simulink library "carnot"  (R2013b)
settings: Solver=ode45  StartTime=0.0  StopTime=10.0  RelTol=1e-3
undefined symbols (not defined in the file or in its folder): A, acol, Ahabit, Awin, Azimuth_Angle, AziWin, B, C, c1, c4, capc, caph, CarnotCallbacks_Density, CarnotCallbacks_Enthalpy, CarnotCallbacks_Enthalpy2Temperature, CarnotCallbacks_Entropy, CarnotCallbacks_Evaporation_Enthalpy, CarnotCallbacks_GlobalMessageLevel, CarnotCallbacks_Grashof, CarnotCallbacks_Heat_Capacity, CarnotCallbacks_Kinematic_Viscosity, CarnotCallbacks_Prandtl, CarnotCallbacks_Saturation_Property, CarnotCallbacks_Saturation_Temperature, CarnotCallbacks_Saturation_Value_Water, CarnotCallbacks_Specific_Volume, CarnotCallbacks_Thermal_Conductivity, CarnotCallbacks_Vapour_Content, CarnotCallbacks_Vapour_Pressure, con, cond, d, Dd, density, dfin, dia, DiameterLastPiece, DPConstant, dpipe, DPLinear, DPQuadratic, emission_out, fluid, FluidMix, FluidType, FPC, frame, g, GeodeticHeight, Gwin, heat_capacity, hgt, HP, Hroom, ID, inlet, K, l, lin, lpipe ... (+29)
undefined symbols (not defined in the file): c2, c3, c5, c6, cwall, dactive, height, mc, mID, rho, tau, UAneighbour, UAwall, uloss
libraries: carnot x333, simulink x25, simulink_extras x7
(part 15 of 16)

== system carnot/Source/Ventilation/Ventilation_AIV/Subsystem ==
  note: (kg/s)
  note: (kg/s)
  note: (kg/s)
  note: (kg/kg)
  note: (kg/kg)
  note: ASSUMPTION: mdot_air_out2in = mdot_air_in2out !
  mdot_air : Inport
  x_in : Inport  Port=2
  x_out : Inport  Port=3
  Demux2 : Demux  Outputs=2
  Demux3 : Demux  Outputs=2
  Fcn{,1..3} (4 alike) : Fcn  Expr=u / (1+u)
  Product5 : Product  SaturateOnIntegerOverflow=on  InputSameDT=on  OutDataTypeStr=Inherit: Same as first input
  Product6 : Product  SaturateOnIntegerOverflow=on  InputSameDT=on  OutDataTypeStr=Inherit: Same as first input
  Sum1 : Sum  Inputs=+-  SaturateOnIntegerOverflow=on  InputSameDT=on  OutDataTypeStr=Inherit: Same as first input
  Sum2 : Sum  Inputs=+-  SaturateOnIntegerOverflow=on  InputSameDT=on  OutDataTypeStr=Inherit: Same as first input
  mdot_H2O : Outport
  mdot_CO2 : Outport  Port=2
  wires:
  x_out/1 -> Demux2/1
  Demux2/1 -> Fcn/1  "x_H2O_out"
  Demux2/2 -> Fcn1/1  "x_CO2_out"
  Demux3/2 -> Fcn3/1  "x_CO2_in"
  Demux3/1 -> Fcn2/1  "x_H2O_in"
  x_in/1 -> Demux3/1
  Fcn/1 -> Sum1/1
  Fcn2/1 -> Sum1/2
  Fcn1/1 -> Sum2/1
  Fcn3/1 -> Sum2/2
  Sum2/1 -> Product6/2
  Sum1/1 -> Product5/2
  mdot_air/1 -> Product6/1, Product5/1  "mdot_air >=0"
  Product6/1 -> mdot_CO2/1
  Product5/1 -> mdot_H2O/1

== system carnot/Storage/Thermal/Storage_Ports/Electric_Heating ==
  electric power : Inport
  Gain : Gain  Gain=Q
  Mux3 : Mux  Inputs=8
  T_in : Constant  Value=ones(nodes,1)*20
  const2 : Constant  Value=1e5
  const3 : Constant
  const4 : Constant  Value=0
  mdot : Constant  Value=zeros(nodes,1)
  to_storeT : Outport
  wires:
  const3/1 -> Mux3/7
  const2/1 -> Mux3/6
  mdot/1 -> Mux3/2, Mux3/3, Mux3/4  "mdot_in"
  Mux3/1 -> to_storeT/1
  T_in/1 -> Mux3/1  "T_in"
  electric power/1 -> Gain/1
  const4/1 -> Mux3/8
  Gain/1 -> Mux3/5  "Qdot_in"

== system carnot/Storage/Thermal/Storage_Ports/HX_EN12977 ==
  from_storeT : Inport
  THBin : Inport  Port=2
  Bus Assignment1 : BusAssignment  AssignedSignals=Temperature
  Mux3 : Mux  Inputs=8
  Pressure_Drop_StorageHX : carnot/Basic/Pressure_Drop/Pressure_Drop_StorageHX  dia=dia  hgt=hgt
  T_in : Constant  Value=zeros(nodes,1)
  fluid : Constant  Value=-9999
  mdot_in : Constant  Value=zeros(nodes,1)
  mix : Constant  Value=-9999
  p : Constant  Value=-9999
  select_Tout : Selector  InputPortWidth=nodes  IndexOptions=Index vector (dialog)  Indices=[outlet]  OutputSizes=1
  sfun_storage_heatexchanger : carnot/Basic/Thermal_Models/sfun_storage_heatexchanger  idn=heat transfer data fit EN12977  nodes=nodes  inlet=inlet  outlet=outlet  pp=[ua0, uam, uat, 0,0,0,0]
  to_storeT : Outport  InitialOutput=0
  THBout : Outport  Port=2  InitialOutput=0
  wires:
  from_storeT/1 -> sfun_storage_heatexchanger/1
  THBin/1 -> Pressure_Drop_StorageHX/1, sfun_storage_heatexchanger/2
  mdot_in/1 -> Mux3/2, Mux3/3, Mux3/4  "mdot_in"
  Mux3/1 -> to_storeT/1
  select_Tout/1 -> Bus Assignment1/2
  T_in/1 -> Mux3/1  "T_in"
  sfun_storage_heatexchanger/1 -> Mux3/5  "Q_in"
  Bus Assignment1/1 -> THBout/1
  p/1 -> Mux3/6
  fluid/1 -> Mux3/7
  mix/1 -> Mux3/8
  sfun_storage_heatexchanger/2 -> select_Tout/1
  Pressure_Drop_StorageHX/1 -> Bus Assignment1/1

== system carnot/Storage/Thermal/Storage_Ports/HX_EN12977_stratified ==
  from_storeT : Inport
  THBin : Inport  Port=2
  Bus Assignment1 : BusAssignment  AssignedSignals=Temperature
  Mux3 : Mux  Inputs=8
  Pressure_Drop_StorageHX : carnot/Basic/Pressure_Drop/Pressure_Drop_StorageHX  dia=dia  hgt=hgt
  T_in : Constant  Value=zeros(nodes,1)
  fluid : Constant  Value=-9999
  mdot_in : Constant  Value=zeros(nodes,1)
  mix : Constant  Value=-9999
  p : Constant  Value=-9999
  select_Tout : Selector  InputPortWidth=nodes  IndexOptions=Index vector (dialog)  Indices=[outlet]  OutputSizes=1
  sfun_storage_heatexchanger : carnot/Basic/Thermal_Models/sfun_storage_heatexchanger  idn="heat transfer data fit EN12977  - stratified"  nodes=nodes  inlet=inlet  outlet=outlet  pp=[ua0, uam, uat, 0,0,0,0]
  to_storeT : Outport  InitialOutput=0
  THBout : Outport  Port=2  InitialOutput=0
  wires:
  from_storeT/1 -> sfun_storage_heatexchanger/1
  THBin/1 -> Pressure_Drop_StorageHX/1, sfun_storage_heatexchanger/2
  mdot_in/1 -> Mux3/2, Mux3/3, Mux3/4  "mdot_in"
  Mux3/1 -> to_storeT/1
  select_Tout/1 -> Bus Assignment1/2
  T_in/1 -> Mux3/1  "T_in"
  sfun_storage_heatexchanger/1 -> Mux3/5  "Q_in"
  Bus Assignment1/1 -> THBout/1
  p/1 -> Mux3/6
  fluid/1 -> Mux3/7
  mix/1 -> Mux3/8
  sfun_storage_heatexchanger/2 -> select_Tout/1
  Pressure_Drop_StorageHX/1 -> Bus Assignment1/1

== system carnot/Storage/Thermal/Storage_Ports/HX_data_fit ==
  note: UA = uac + mdot*uam + (Thx-Tstorage)*uat
      | Qdot = UA * (Tstore-Thx)
  from_storeT : Inport
  THBin : Inport  Port=2
  Bus Assignment1 : BusAssignment  AssignedSignals=Temperature
  Mux3 : Mux  Inputs=8
  Pressure_Drop_StorageHX : carnot/Basic/Pressure_Drop/Pressure_Drop_StorageHX  dia=dia  hgt=hgt
  T_in : Constant  Value=zeros(nodes,1)
  fluid : Constant  Value=-9999
  mdot_in : Constant  Value=zeros(nodes,1)
  mix : Constant  Value=-9999
  p : Constant  Value=-9999
  select_Tout : Selector  InputPortWidth=nodes  IndexOptions=Index vector (dialog)  Indices=[outlet]  OutputSizes=1
  sfun_storage_heatexchanger : carnot/Basic/Thermal_Models/sfun_storage_heatexchanger  idn=heat transfer from data fit  nodes=nodes  inlet=inlet  outlet=outlet  pp=[ua0, uam, uat, 0,0,0,0]
  to_storeT : Outport
  THBout : Outport  Port=2
  wires:
  sfun_storage_heatexchanger/2 -> select_Tout/1
  mix/1 -> Mux3/8
  fluid/1 -> Mux3/7
  p/1 -> Mux3/6
  Bus Assignment1/1 -> THBout/1
  sfun_storage_heatexchanger/1 -> Mux3/5  "Q_in"
  T_in/1 -> Mux3/1  "T_in"
  select_Tout/1 -> Bus Assignment1/2
  Mux3/1 -> to_storeT/1
  mdot_in/1 -> Mux3/4, Mux3/3, Mux3/2  "mdot_in"
  THBin/1 -> Pressure_Drop_StorageHX/1, sfun_storage_heatexchanger/2
  from_storeT/1 -> sfun_storage_heatexchanger/1
  Pressure_Drop_StorageHX/1 -> Bus Assignment1/1

== system carnot/Storage/Thermal/Storage_Ports/HX_data_fit_stratified ==
  note: statified charging !
      | heat transfer:
      | UA = uac + mdot*uam + (Thx-Tstorage)*uat
      | Qdot = UA * (Tstore-Thx)
  from_storeT : Inport
  THBin : Inport  Port=2
  Bus Assignment1 : BusAssignment  AssignedSignals=Temperature
  Mux3 : Mux  Inputs=8
  Pressure_Drop_StorageHX : carnot/Basic/Pressure_Drop/Pressure_Drop_StorageHX  dia=dia  hgt=hgt
  T_in : Constant  Value=zeros(nodes,1)
  fluid : Constant  Value=-9999
  mdot_in : Constant  Value=zeros(nodes,1)
  mix : Constant  Value=-9999
  p : Constant  Value=-9999
  select_Tout : Selector  InputPortWidth=nodes  IndexOptions=Index vector (dialog)  Indices=[outlet]  OutputSizes=1
  sfun_storage_heatexchanger : carnot/Basic/Thermal_Models/sfun_storage_heatexchanger  idn="heat transfer from data fit  - stratified"  nodes=nodes  inlet=inlet  outlet=outlet  pp=[ua0, uam, uat, 0,0,0,0]
  to_storeT : Outport  InitialOutput=0
  THBout : Outport  Port=2  InitialOutput=0
  wires:
  from_storeT/1 -> sfun_storage_heatexchanger/1
  THBin/1 -> Pressure_Drop_StorageHX/1, sfun_storage_heatexchanger/2
  mdot_in/1 -> Mux3/2, Mux3/3, Mux3/4  "mdot_in"
  Mux3/1 -> to_storeT/1
  select_Tout/1 -> Bus Assignment1/2
  T_in/1 -> Mux3/1  "T_in"
  sfun_storage_heatexchanger/1 -> Mux3/5  "Q_in"
  p/1 -> Mux3/6
  fluid/1 -> Mux3/7
  mix/1 -> Mux3/8
  sfun_storage_heatexchanger/2 -> select_Tout/1
  Pressure_Drop_StorageHX/1 -> Bus Assignment1/1
  Bus Assignment1/1 -> THBout/1

== system carnot/Storage/Thermal/Storage_Ports/HX_finned_tube ==
  from_storeT : Inport
  THBin : Inport  Port=2
  Bus Assignment1 : BusAssignment  AssignedSignals=Temperature
  Mux3 : Mux  Inputs=8
  Pressure_Drop_StorageHX : carnot/Basic/Pressure_Drop/Pressure_Drop_StorageHX  dia=dia  hgt=hgt
  T_in : Constant  Value=zeros(nodes,1)
  fluid : Constant  Value=-9999
  mdot_in : Constant  Value=zeros(nodes,1)
  mix : Constant  Value=-9999
  p : Constant  Value=-9999
  select_Tout : Selector  InputPortWidth=nodes  IndexOptions=Index vector (dialog)  Indices=[outlet]  OutputSizes=1
  sfun_storage_heatexchanger : carnot/Basic/Thermal_Models/sfun_storage_heatexchanger  idn=finned tube theoretical  nodes=nodes  inlet=inlet  outlet=outlet  pp=[dpipe, swall, lpipe, cond, dfin, sfin, nfin]
  to_storeT : Outport  InitialOutput=0
  THBout : Outport  Port=2  InitialOutput=0
  wires:
  from_storeT/1 -> sfun_storage_heatexchanger/1
  THBin/1 -> Pressure_Drop_StorageHX/1, sfun_storage_heatexchanger/2
  mdot_in/1 -> Mux3/2, Mux3/3, Mux3/4  "mdot_in"
  Mux3/1 -> to_storeT/1
  select_Tout/1 -> Bus Assignment1/2
  T_in/1 -> Mux3/1  "T_in"
  sfun_storage_heatexchanger/1 -> Mux3/5  "Q_in"
  Bus Assignment1/1 -> THBout/1
  p/1 -> Mux3/6
  fluid/1 -> Mux3/7
  mix/1 -> Mux3/8
  sfun_storage_heatexchanger/2 -> select_Tout/1
  Pressure_Drop_StorageHX/1 -> Bus Assignment1/1

== system carnot/Storage/Thermal/Storage_Ports/HX_finned_tube_stratified ==
  from_storeT : Inport
  THBin : Inport  Port=2
  Bus Assignment1 : BusAssignment  AssignedSignals=Temperature
  Mux3 : Mux  Inputs=8
  Pressure_Drop_StorageHX : carnot/Basic/Pressure_Drop/Pressure_Drop_StorageHX  dia=dia  hgt=hgt
  T_in : Constant  Value=zeros(nodes,1)
  fluid : Constant  Value=-9999
  mdot_in : Constant  Value=zeros(nodes,1)
  mix : Constant  Value=-9999
  p : Constant  Value=-9999
  select_Tout : Selector  InputPortWidth=nodes  IndexOptions=Index vector (dialog)  Indices=[outlet]  OutputSizes=1
  sfun_storage_heatexchanger : carnot/Basic/Thermal_Models/sfun_storage_heatexchanger  idn="finned tube theoretical  - stratified"  nodes=nodes  inlet=inlet  outlet=outlet  pp=[dpipe, swall, lpipe, cond, dfin, sfin, nfin]
  to_storeT : Outport  InitialOutput=0
  THBout : Outport  Port=2  InitialOutput=0
  wires:
  Pressure_Drop_StorageHX/1 -> Bus Assignment1/1
  sfun_storage_heatexchanger/2 -> select_Tout/1
  mix/1 -> Mux3/8
  fluid/1 -> Mux3/7
  p/1 -> Mux3/6
  Bus Assignment1/1 -> THBout/1
  sfun_storage_heatexchanger/1 -> Mux3/5  "Q_in"
  T_in/1 -> Mux3/1  "T_in"
  select_Tout/1 -> Bus Assignment1/2
  Mux3/1 -> to_storeT/1
  mdot_in/1 -> Mux3/4, Mux3/3, Mux3/2  "mdot_in"
  THBin/1 -> sfun_storage_heatexchanger/2, Pressure_Drop_StorageHX/1
  from_storeT/1 -> sfun_storage_heatexchanger/1

== system carnot/Storage/Thermal/Storage_Ports/HX_tube ==
  from_storeT : Inport
  THBin : Inport  Port=2
  Bus Assignment1 : BusAssignment  AssignedSignals=Temperature
  Mux3 : Mux  Inputs=8
  Pressure_Drop_StorageHX : carnot/Basic/Pressure_Drop/Pressure_Drop_StorageHX  dia=dia  hgt=hgt
  T_in : Constant  Value=zeros(nodes,1)
  fluid : Constant  Value=-9999
  mdot_in : Constant  Value=zeros(nodes,1)
  mix : Constant  Value=-9999
  p : Constant  Value=-9999
  select_Tout : Selector  InputPortWidth=nodes  IndexOptions=Index vector (dialog)  Indices=[outlet]  OutputSizes=1
  sfun_storage_heatexchanger : carnot/Basic/Thermal_Models/sfun_storage_heatexchanger  idn=smooth tube theoretical  nodes=nodes  inlet=inlet  outlet=outlet  pp=[dpipe, swall, lpipe, cond, 0,0,0]
  to_storeT : Outport  InitialOutput=0
  THBout : Outport  Port=2  InitialOutput=0
  wires:
  Pressure_Drop_StorageHX/1 -> Bus Assignment1/1
  sfun_storage_heatexchanger/2 -> select_Tout/1
  mix/1 -> Mux3/8
  fluid/1 -> Mux3/7
  p/1 -> Mux3/6
  Bus Assignment1/1 -> THBout/1
  sfun_storage_heatexchanger/1 -> Mux3/5  "Q_in"
  T_in/1 -> Mux3/1  "T_in"
  select_Tout/1 -> Bus Assignment1/2
  Mux3/1 -> to_storeT/1
  mdot_in/1 -> Mux3/4, Mux3/3, Mux3/2  "mdot_in"
  THBin/1 -> Pressure_Drop_StorageHX/1, sfun_storage_heatexchanger/2
  from_storeT/1 -> sfun_storage_heatexchanger/1

== system carnot/Storage/Thermal/Storage_Ports/HX_tube_stratified ==
  from_storeT : Inport
  THBin : Inport  Port=2
  Bus Assignment1 : BusAssignment  AssignedSignals=Temperature
  Mux3 : Mux  Inputs=8
  Pressure_Drop_StorageHX : carnot/Basic/Pressure_Drop/Pressure_Drop_StorageHX  dia=dia  hgt=hgt
  T_in : Constant  Value=zeros(nodes,1)
  fluid : Constant  Value=-9999
  mdot_in : Constant  Value=zeros(nodes,1)
  mix : Constant  Value=-9999
  p : Constant  Value=-9999
  select_Tout : Selector  InputPortWidth=nodes  IndexOptions=Index vector (dialog)  Indices=[outlet]  OutputSizes=1
  sfun_storage_heatexchanger : carnot/Basic/Thermal_Models/sfun_storage_heatexchanger  idn=smooth tube theoretical - stratified  nodes=nodes  inlet=inlet  outlet=outlet  pp=[dpipe, swall, lpipe, cond, 0,0,0]
  to_storeT : Outport  InitialOutput=0
  THBout : Outport  Port=2  InitialOutput=0
  wires:
  Pressure_Drop_StorageHX/1 -> Bus Assignment1/1
  sfun_storage_heatexchanger/2 -> select_Tout/1
  mix/1 -> Mux3/8
  fluid/1 -> Mux3/7
  p/1 -> Mux3/6
  Bus Assignment1/1 -> THBout/1
  sfun_storage_heatexchanger/1 -> Mux3/5  "Q_in"
  T_in/1 -> Mux3/1  "T_in"
  select_Tout/1 -> Bus Assignment1/2
  Mux3/1 -> to_storeT/1
  mdot_in/1 -> Mux3/4, Mux3/3, Mux3/2  "mdot_in"
  THBin/1 -> Pressure_Drop_StorageHX/1, sfun_storage_heatexchanger/2
  from_storeT/1 -> sfun_storage_heatexchanger/1

== system carnot/Storage/Thermal/Storage_Ports/Pipe ==
  from_storeT : Inport
  THBin : Inport  Port=2
  Bus Assignment : BusAssignment  AssignedSignals=Temperature
  Bus Selector : BusSelector  OutputSignals=Temperature,MassFlow,Pressure,FluidType,FluidMix
  Gain : Gain  Gain=in
  Gain1 : Gain  Gain=up
  Gain2 : Gain  Gain=down
  Gain3 : Gain  Gain=in
  Mux3 : Mux  Inputs=8
  Pressure_Drop_StoragePipe : carnot/Basic/Pressure_Drop/Pressure_Drop_StoragePipe  dia=dia  hgt=hgt
  Q_in : Constant  Value=zeros(nodes,1)
  select_Tin_2_Tout : Selector  InputPortWidth=nodes  IndexOptions=Index vector (dialog)  Indices=[idx_in_out]  OutputSizes=1
  select_Tout : Selector  InputPortWidth=nodes  IndexOptions=Index vector (dialog)  Indices=[outlet]  OutputSizes=1
  to_storeT : Outport
  THBout : Outport  Port=2
  wires:
  select_Tin_2_Tout/1 -> Pressure_Drop_StoragePipe/1
  Bus Selector/5 -> Mux3/8  "<FluidMix>"
  Bus Assignment/1 -> THBout/1
  Q_in/1 -> Mux3/5
  Gain3/1 -> Mux3/1  "T_in"
  select_Tout/1 -> Bus Assignment/2
  Mux3/1 -> to_storeT/1
  Gain2/1 -> Mux3/4  "mdot_down"
  Gain1/1 -> Mux3/3  "mdot_up"
  Gain/1 -> Mux3/2  "mdot_in"
  Bus Selector/1 -> Gain3/1  "<Temperature>"
  Bus Selector/2 -> Gain2/1, Gain1/1, Gain/1  "<MassFlow>"
  Bus Selector/3 -> Mux3/6  "<Pressure>"
  Bus Selector/4 -> Mux3/7  "<FluidType>"
  THBin/1 -> Bus Selector/1, Pressure_Drop_StoragePipe/2
  from_storeT/1 -> select_Tin_2_Tout/1, select_Tout/1
  Pressure_Drop_StoragePipe/1 -> Bus Assignment/1

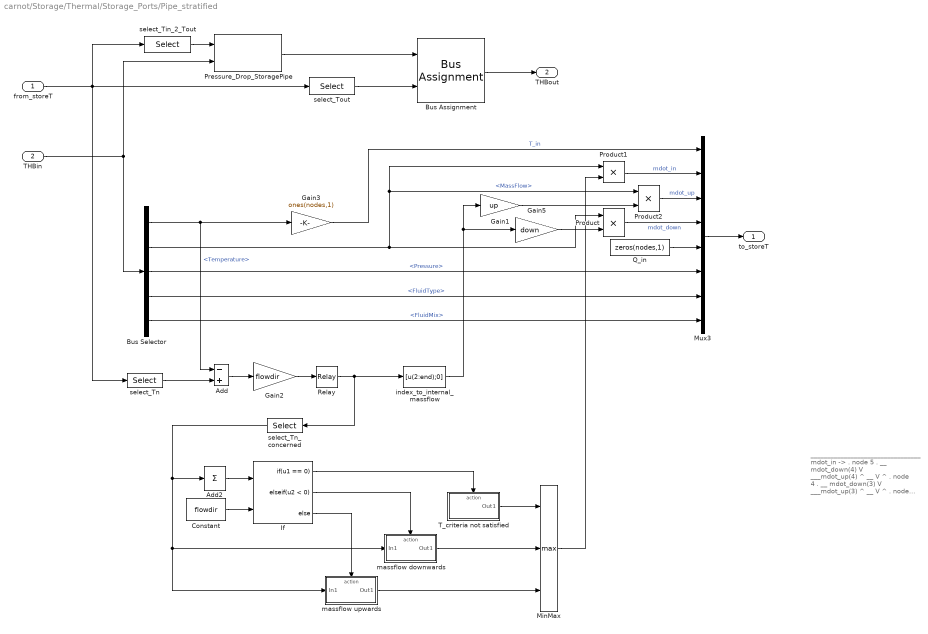
== system carnot/Storage/Thermal/Storage_Ports/Pipe_stratified ==
  note: _________________________________
      | mdot_in ->                                                .
      | node 5                     .
      | __ mdot_down(4) V  ___mdot_up(4) ^ __
      | V                           ^    .
      | node 4                    .
      | __ mdot_down(3) V  ___mdot_up(3) ^ __
      | V                           ^    .
      | node 3                    .
      | __ mdot_down(2) V  ___mdot_up(2) ^ __
      | V                           ^    .
      | node 2                    .
      | __ mdot_down(1) V  ___mdot_up(1) ^ __
      | V                           ^    .
      | node 1                    .
      | _________________________________
  from_storeT : Inport
  THBin : Inport  Port=2
  Add : Sum  Inputs=-+
  Add2 : Sum  Inputs=1
  Bus Assignment : BusAssignment  AssignedSignals=Temperature
  Bus Selector : BusSelector  OutputSignals=Temperature,MassFlow,Pressure,FluidType,FluidMix
  Constant : Constant  Value=flowdir
  Gain1 : Gain  Gain=up
  Gain2 : Gain  Gain=flowdir
  Gain3 : Gain  Gain=ones(nodes,1)
  Gain5 : Gain  Gain=down
  If : If  NumInputs=2  IfExpression=u1 == 0  ElseIfExpressions=u2 < 0
  MinMax : MinMax  Function=max  Inputs=3
  Mux3 : Mux  Inputs=8
  Pressure_Drop_StoragePipe : carnot/Basic/Pressure_Drop/Pressure_Drop_StoragePipe  dia=dia  hgt=hgt
  Product : Product  RndMeth=Zero
  Product1 : Product  RndMeth=Zero
  Product2 : Product  RndMeth=Zero
  Q_in : Constant  Value=zeros(nodes,1)
  Relay : Relay  OnSwitchValue=0.05  OffSwitchValue=-0.05
  T_criteria not satisfied : Subsystem  TreatAsAtomicUnit=on
  index_to_internal_massflow : MATLABFcn  MATLABFcn=[u(2:end);0]  OutputDimensions=nodes
  massflow downwards : Subsystem  TreatAsAtomicUnit=on
  massflow upwards : Subsystem  TreatAsAtomicUnit=on
  select_Tin_2_Tout : Selector  InputPortWidth=nodes  IndexOptions=Index vector (dialog)  Indices=[idx_in_out]  OutputSizes=1
  select_Tn : Selector  InputPortWidth=nodes  IndexOptions=Index vector (dialog)  Indices=[1:nodes]  OutputSizes=1
  select_Tn_concerned : Selector  InputPortWidth=nodes  IndexOptions=Index vector (dialog)  Indices=n_concerned  OutputSizes=1
  select_Tout : Selector  InputPortWidth=nodes  IndexOptions=Index vector (dialog)  Indices=[outlet]  OutputSizes=1
  to_storeT : Outport
  THBout : Outport  Port=2
  wires:
  select_Tin_2_Tout/1 -> Pressure_Drop_StoragePipe/1
  Pressure_Drop_StoragePipe/1 -> Bus Assignment/1
  select_Tn_concerned/1 -> Add2/1, massflow downwards/1(In1), massflow upwards/1(In1)
  MinMax/1 -> Product1/2
  Add2/1 -> If/1
  Product1/1 -> Mux3/2  "mdot_in"
  Gain5/1 -> Product/2
  Relay/1 -> select_Tn_concerned/1, index_to_internal_massflow/1
  Product/1 -> Mux3/4  "mdot_down"
  from_storeT/1 -> select_Tin_2_Tout/1, select_Tn/1, select_Tout/1
  THBin/1 -> Pressure_Drop_StoragePipe/2, Bus Selector/1
  Bus Selector/4 -> Mux3/7  "<FluidType>"
  Bus Selector/3 -> Mux3/6  "<Pressure>"
  Bus Selector/2 -> Product/1, Product2/1, Product1/1  "<MassFlow>"
  Bus Selector/1 -> Gain3/1, Add/1  "<Temperature>"
  Mux3/1 -> to_storeT/1
  select_Tout/1 -> Bus Assignment/2
  Gain3/1 -> Mux3/1  "T_in"
  Q_in/1 -> Mux3/5
  Bus Assignment/1 -> THBout/1
  Bus Selector/5 -> Mux3/8  "<FluidMix>"
  select_Tn/1 -> Add/2
  Add/1 -> Gain2/1
  If/1 -> T_criteria not satisfied/Action
  Constant/1 -> If/2
  T_criteria not satisfied/1(Out1) -> MinMax/1
  If/2 -> massflow downwards/Action
  If/3 -> massflow upwards/Action
  massflow downwards/1(Out1) -> MinMax/2
  Gain1/1 -> Product2/2
  Product2/1 -> Mux3/3  "mdot_up"
  massflow upwards/1(Out1) -> MinMax/3
  Gain2/1 -> Relay/1
  index_to_internal_massflow/1 -> Gain5/1, Gain1/1

== system carnot/Storage/Thermal/detailed_storage_models/heat_exchanger_storage ==
  Tamb : Inport
  THVex_in : Inport  Port=2
  THVstg_in : Inport  Port=3
  Demux : Demux
  Demux1 : Demux  Outputs=[1 1 1 1 2]
  Demux2 : Demux  Outputs=[1 1 1 1 2]
  Demux3 : Demux  Outputs=[6 14]
  Demux4 : Demux  Outputs=[6 14]
  Mux : Mux  Inputs=11
  Mux1 : Mux  Inputs=6
  Mux2 : Mux  Inputs=6
  S-Function : S-Function  FunctionName=ministg  Parameters=v(1), v(2), loss, uh(1), uh(2), uc(1), uc(2), uw(1), uw(2), mat, m(1), m(2), t0, dph(1), dph(2), dph(3), dpc(1), dpc(2), dpc(3), n  EnableBusSupport=off
  THVex : Outport
  THVstg : Outport  Port=2
  wires:
  Demux2/5 -> Mux2/5, Mux/11  "fluid, mix"
  Demux2/3 -> Mux2/3, Mux/9  "mdot"
  Demux1/5 -> Mux1/5, Mux/6  "fluid, mix"
  Demux1/3 -> Mux1/3, Mux/4  "mdot"
  Demux1/4 -> Mux/5
  Demux1/2 -> Mux/3
  Mux/1 -> S-Function/1
  Tamb/1 -> Mux/1
  Demux1/1 -> Mux1/1, Mux/2  "ID"
  Demux2/4 -> Mux/10
  Demux2/2 -> Mux/8
  Demux2/1 -> Mux2/1, Mux/7  "ID"
  S-Function/1 -> Demux/1
  Demux3/1 -> Demux1/1
  THVex_in/1 -> Demux3/1
  THVstg_in/1 -> Demux4/1
  Demux4/1 -> Demux2/1
  Demux/4 -> Mux2/4
  Demux/3 -> Mux2/2
  Mux2/1 -> THVstg/1
  Mux1/1 -> THVex/1
  Demux/2 -> Mux1/4
  Demux/1 -> Mux1/2
  Demux3/2 -> Mux1/6
  Demux4/2 -> Mux2/6

== system carnot/Storage/Thermal/surface_models/Isolated_Cover ==
  Tamb : Inport
  Mux2 : Mux  Inputs=2
  const1 : Constant  Value=[u 0]
  Tamb_utop_Iabs : Outport
  wires:
  Mux2/1 -> Tamb_utop_Iabs/1
  const1/1 -> Mux2/2
  Tamb/1 -> Mux2/1

== system carnot/Storage/Thermal/surface_models/Open_Surface ==
  WDB : Inport
  3*vwind : Gain  Gain=3  SaturateOnIntegerOverflow=on  OutDataTypeStr=Inherit: Same as input  ParamDataTypeStr=Inherit: Same as input
  Bus Selector : BusSelector  OutputSignals=Solar_Radiation_direct_surface,Solar_Radiation_diffuse_surface,Temperature_Ambient,Wind_Speed
  Fixed_Surface : carnot/Weather/Fixed_Surface  colangle=0  colazi=0  colrot=0
  Mux2 : Mux  Inputs=3
  Radiation_on_Inclined_Surface : carnot/Weather/Radiation_on_Inclined_Surface  sky=Perez 1990  reflect=0.2
  Sum : Sum  Inputs=2  SaturateOnIntegerOverflow=on  InputSameDT=on  OutDataTypeStr=Inherit: Same as first input
  add 5.6 : Subsystem  mask(add constant){c=5.6}
      mask prompts: c "constant c"
      mask help: This block adds a constant c to each element of the input vector.
      mask Help: file:///constant.htm
      mask Display: disp('+c');
  ground absorbtion : Gain  Gain=albedo  SaturateOnIntegerOverflow=on  OutDataTypeStr=Inherit: Same as input  ParamDataTypeStr=Inherit: Same as input
  Tamb_utop_Iabs : Outport
  wires:
  Bus Selector/2 -> Sum/2  "<Solar_Radiation_diffuse_surface>"
  WDB/1 -> Radiation_on_Inclined_Surface/1
  Fixed_Surface/1 -> Radiation_on_Inclined_Surface/2
  Radiation_on_Inclined_Surface/1 -> Bus Selector/1
  Bus Selector/3 -> Mux2/1  "<Temperature_Ambient>"
  ground absorbtion/1 -> Mux2/3
  Bus Selector/1 -> Sum/1  "<Solar_Radiation_direct_surface>"
  Sum/1 -> ground absorbtion/1
  3*vwind/1 -> add 5.6/1(In1)
  add 5.6/1(Out1) -> Mux2/2
  Mux2/1 -> Tamb_utop_Iabs/1
  Bus Selector/4 -> 3*vwind/1  "<Wind_Speed>"

== system carnot/Basic/Thermal_Models/Combustion_Calculation/exhaust gas/fluid//solid ==
  c : Inport
  h : Inport  Port=2
  s : Inport  Port=3
  n : Inport  Port=4
  w : Inport  Port=5
  Mux : Mux  Inputs=2
  Mux1 : Mux
  kgCO2 : Gain  Gain=3.67  SaturateOnIntegerOverflow=on  OutDataTypeStr=Inherit: Same as input  ParamDataTypeStr=Inherit: Same as input
  kgH2O : Fcn  Expr=9*u(1)+u(2)
  kgSO2 : Gain  Gain=2  SaturateOnIntegerOverflow=on  OutDataTypeStr=Inherit: Same as input  ParamDataTypeStr=Inherit: Same as input
  Out1 : Outport
  wires:
  n/1 -> Mux1/4
  s/1 -> kgSO2/1
  w/1 -> Mux/2
  Mux1/1 -> Out1/1
  h/1 -> Mux/1
  c/1 -> kgCO2/1
  kgSO2/1 -> Mux1/3
  kgH2O/1 -> Mux1/2
  kgCO2/1 -> Mux1/1
  Mux/1 -> kgH2O/1

== system carnot/Basic/Thermal_Models/Combustion_Calculation/exhaust gas/gas ==
  c : Inport
  h : Inport  Port=2
  s : Inport  Port=3
  n : Inport  Port=4
  Mux1 : Mux
  Terminator1 : Terminator
  kgCO2 : Gain  Gain=3.67  SaturateOnIntegerOverflow=on  OutDataTypeStr=Inherit: Same as input  ParamDataTypeStr=Inherit: Same as input
  kgH2O : Gain  Gain=9  SaturateOnIntegerOverflow=on  OutDataTypeStr=Inherit: Same as input  ParamDataTypeStr=Inherit: Same as input
  kgSO2 : Ground
  Out1 : Outport
  wires:
  n/1 -> Mux1/4
  kgSO2/1 -> Mux1/3
  kgH2O/1 -> Mux1/2
  kgCO2/1 -> Mux1/1
  Mux1/1 -> Out1/1
  s/1 -> Terminator1/1
  h/1 -> kgH2O/1
  c/1 -> kgCO2/1

== system carnot/Basic/Thermal_Models/HeatPump_basic/model cold side/add constant ==
  In1 : Inport
  Sum : Sum  SaturateOnIntegerOverflow=on  InputSameDT=on  OutDataTypeStr=Inherit: Same as first input
  const : Constant  Value=c
  Out1 : Outport
  wires:
  const/1 -> Sum/1
  In1/1 -> Sum/2
  Sum/1 -> Out1/1

== system carnot/Load/Houses/heat_transfer/alfa_wall_out/q rad ==
  note: Wall has a view on 50% ground and 50% sky (true for vertical walls).
      | Longwave radiation emissiviy of ground and sky assumed to be 1.
  Tamb : Inport
  Twall : Inport  Port=2
  Tsky : Inport  Port=3
  Bias : Bias  Bias=273.15
  Gain : Gain  Gain=[-1 0.5 0.5]*emission_out*5.67e-8
  Math Function : Math  Operator=square  SaturateOnIntegerOverflow=on
  Math Function1 : Math  Operator=square  SaturateOnIntegerOverflow=on
  Mux : Mux  Inputs=3
  Sum : Sum  Inputs=1  SaturateOnIntegerOverflow=on  InputSameDT=on  OutDataTypeStr=Inherit: Same as first input
  qrad : Outport
  wires:
  Math Function1/1 -> Gain/1
  Gain/1 -> Sum/1
  Math Function/1 -> Math Function1/1
  Mux/1 -> Bias/1
  Bias/1 -> Math Function/1
  Twall/1 -> Mux/1
  Sum/1 -> qrad/1
  Tamb/1 -> Mux/3
  Tsky/1 -> Mux/2

== system carnot/Load/Houses/heat_transfer/alfa_window_in/Irradiation into room ==
  note: Solar radiation into zone
  "[tau]" : Inport
  "[I_t]" : Inport  Port=2
  Dot Product : DotProduct  InputSameDT=on  OutDataTypeStr=Inherit: Inherit via internal rule
  Selector : Selector  InputPortWidth=3  IndexOptions=Index vector (dialog)  Indices=[1 3]  OutputSizes=1
  Sum2 : Sum  Inputs=1  SaturateOnIntegerOverflow=on  InputSameDT=on  OutDataTypeStr=Inherit: Same as first input
  const : Gain  Gain=gvalue  SaturateOnIntegerOverflow=on  OutDataTypeStr=Inherit: Same as input  ParamDataTypeStr=Inherit: Same as input
  qdot_sol : Outport
  wires:
  const/1 -> qdot_sol/1
  Sum2/1 -> const/1
  Dot Product/1 -> Sum2/1
  Selector/1 -> Dot Product/1
  "[tau]"/1 -> Selector/1  "tau_dir(teta), tau_dir(0), tau_dfu"
  "[I_t]"/1 -> Dot Product/2

== system carnot/Load/Houses/heat_transfer/alfa_window_in/transmission coefficient 1-2-3-4-layer(s) ==
  teta : Inport
  LUT_taualfa : Subsystem  mask(LOOK UP TABLE){}
      mask help:
      | This block delivers the standardized LIGHT TRANSMISSION COEFFICIENT of a window glass with 1, 2, 3 or 4 layers depending on the incidence angle. Each layer may be 3 to 8 mm thick.
      |
      | teta:    incidence angle = angle between surface normal and
      |                 incidence, degree
      | numlayer: number of layers within the window glass, [1,4].
      | tau:    transmission of glass layer stack, [0,1]
  Mux : Mux  Inputs=3
  numlayer : Constant  Value=numlayer
  perpendicular : Constant  Value=0
  tau,dfu - angle : Constant  Value=60
  "[tau]" : Outport
  wires:
  LUT_taualfa/1(tau) -> "[tau]"/1
  numlayer/1 -> LUT_taualfa/2(numlayer)
  Mux/1 -> LUT_taualfa/1(teta)
  perpendicular/1 -> Mux/2
  tau,dfu - angle/1 -> Mux/3
  teta/1 -> Mux/1

== system carnot/Load/Houses/room_nodes/Room_Node/Sensitive room temperature ==
  note: Sensitive temperature
  Tr : Inport
  Tc : Inport  Port=2
  1-share_c : Gain  Gain=1-share_c  SaturateOnIntegerOverflow=on  OutDataTypeStr=Inherit: Same as input  ParamDataTypeStr=Inherit: Same as input
  Sum : Sum  SaturateOnIntegerOverflow=on  InputSameDT=on  OutDataTypeStr=Inherit: Same as first input
  share_c : Gain  Gain=share_c  SaturateOnIntegerOverflow=on  OutDataTypeStr=Inherit: Same as input  ParamDataTypeStr=Inherit: Same as input
  Ts : Outport
  wires:
  Sum/1 -> Ts/1
  1-share_c/1 -> Sum/2  "Tr"
  share_c/1 -> Sum/1  "Tc"
  Tc/1 -> share_c/1
  Tr/1 -> 1-share_c/1

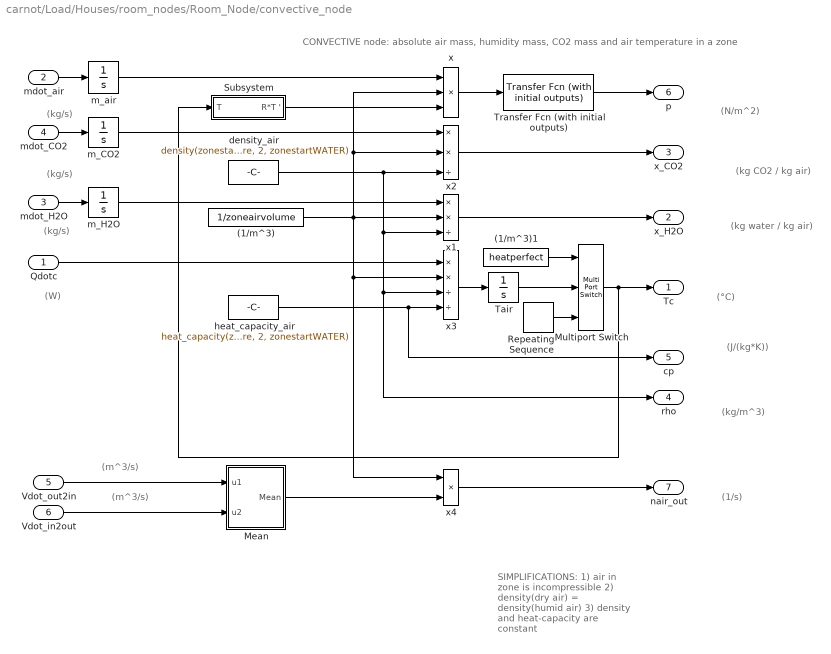
== system carnot/Load/Houses/room_nodes/Room_Node/convective_node ==
  note: (N/m^2)
  note: (kg CO2 / kg air)
  note: (J/(kg*K))
  note: SIMPLIFICATIONS:
      | 1) air in zone is incompressible
      | 2) density(dry air) = density(humid air)
      | 3) density and heat-capacity are constant
  note: (kg/m^3)
  note: CONVECTIVE node: absolute air mass, humidity mass, CO2 mass and air temperature in a zone
  note: (1/s)
  note: (m^3/s)
  note: (kg/s)
  note: (kg/s)
  note: (kg water / kg air)
  note: (°C)
  note: (W)
  note: (kg/s)
  note: (m^3/s)
  Qdotc : Inport
  mdot_air : Inport  Port=2
  mdot_H2O : Inport  Port=3
  mdot_CO2 : Inport  Port=4
  Vdot_out2in : Inport  Port=5
  Vdot_in2out : Inport  Port=6
  (1/m^3) : Constant  Value=1/zoneairvolume
  (1/m^3)1 : Constant  Value=heatperfect
  Mean : Subsystem
  Multiport Switch : MultiPortSwitch  Inputs=2  SaturateOnIntegerOverflow=on  InputSameDT=on
  Repeating Sequence : simulink/Sources/Repeating Sequence  rep_seq_t=lookuptime  rep_seq_y=lookupvalue
  Subsystem : Subsystem
  Tair : Integrator  InitialCondition=zonestartTEMP
  Transfer Fcn (with initial outputs) : simulink_extras/Additional Linear/Transfer Fcn (with initial outputs)  N=[1]  D=[timeconst 1]  Y0=1e5  U0=0
  density_air : Constant  Value=density(zonestartTEMP, AirPressure, 2, zonestartWATER)
  heat_capacity_air : Constant  Value=heat_capacity(zonestartTEMP, AirPressure, 2, zonestartWATER)
  m_CO2 : Integrator  InitialCondition=zonestartCO2  LimitOutput=on  LowerSaturationLimit=0
  m_H2O : Integrator  InitialCondition=zonestartWATER  LimitOutput=on  LowerSaturationLimit=0
  m_air : Integrator  InitialCondition=zonestartAIR  LimitOutput=on  LowerSaturationLimit=0
  x : Product  Inputs=***  SaturateOnIntegerOverflow=on  InputSameDT=on  OutDataTypeStr=Inherit: Same as first input
  x1 : Product  Inputs=**/  SaturateOnIntegerOverflow=on  InputSameDT=on  OutDataTypeStr=Inherit: Same as first input
  x2 : Product  Inputs=**/  SaturateOnIntegerOverflow=on  InputSameDT=on  OutDataTypeStr=Inherit: Same as first input
  x3 : Product  Inputs=**//  SaturateOnIntegerOverflow=on  InputSameDT=on  OutDataTypeStr=Inherit: Same as first input
  x4 : Product  Inputs=**  SaturateOnIntegerOverflow=on  InputSameDT=on  OutDataTypeStr=Inherit: Same as first input
  Tc : Outport
  x_H2O : Outport  Port=2
  x_CO2 : Outport  Port=3
  rho : Outport  Port=4
  cp : Outport  Port=5
  p : Outport  Port=6
  nair_out : Outport  Port=7
  wires:
  Repeating Sequence/1 -> Multiport Switch/3
  (1/m^3)1/1 -> Multiport Switch/1
  Multiport Switch/1 -> Tc/1, Subsystem/1(T)
  x2/1 -> x_CO2/1
  Tair/1 -> Multiport Switch/2
  x3/1 -> Tair/1
  (1/m^3)/1 -> x4/1, x3/2, x1/2, x/2, x2/2
  m_CO2/1 -> x2/1
  heat_capacity_air/1 -> cp/1, x3/4
  m_air/1 -> x/1
  mdot_air/1 -> m_air/1
  Subsystem/1(R*T ') -> x/3
  x1/1 -> x_H2O/1
  mdot_H2O/1 -> m_H2O/1
  mdot_CO2/1 -> m_CO2/1
  m_H2O/1 -> x1/1
  x/1 -> Transfer Fcn (with initial outputs)/1
  x4/1 -> nair_out/1
  Vdot_in2out/1 -> Mean/2(u2)
  Vdot_out2in/1 -> Mean/1(u1)
  Mean/1(Mean) -> x4/2
  Qdotc/1 -> x3/1
  density_air/1 -> x2/3, x1/3, x3/3, rho/1
  Transfer Fcn (with initial outputs)/1 -> p/1

== system carnot/Load/Houses/room_nodes/Room_Node/radiative_node ==
  note: RADIATIVE node
  Qdotr : Inport
  (1/m^3)1 : Constant  Value=heatperfect
  Gain : Gain  Gain=1/timeconst
  Integrator : Integrator  InitialCondition=zonestartTEMP
  Multiport Switch : MultiPortSwitch  Inputs=2  SaturateOnIntegerOverflow=on  InputSameDT=on
  Repeating Sequence : simulink/Sources/Repeating Sequence  rep_seq_t=lookuptime  rep_seq_y=lookupvalue
  Tr : Outport
  wires:
  Repeating Sequence/1 -> Multiport Switch/3
  Gain/1 -> Integrator/1
  Qdotr/1 -> Gain/1
  (1/m^3)1/1 -> Multiport Switch/1
  Integrator/1 -> Multiport Switch/2
  Multiport Switch/1 -> Tr/1

== system carnot/Load/Houses/wall_floor/Window_with_Shading/alfa_window_in ==
  note: (W/m^2)
  note: CONVENTION:
      | Qdot > 0 and qdots < 0, if Ts > T (heat flows from wall surface to room node),
      | Qdot < 0 and qdots > 0, if Ts < T (heat flows from room node to wall surface).
  note: s: surface
      | c: convective
      | r: radiative
  note: WINDOW = FRAME + GLASS
  note: Convective and radiative heat transfer at the INDOOR SURFACE OF A VERTICAL WINDOW
      | with 1-4 layers (each 3 ... 8 mm thick)
  note: (°C)
  Ts2 : Inport
  "[sun_t]" : Inport  Port=2
  "[AIV]" : Inport  Port=3
  WDB : Inport  Port=4
  control : Inport  Port=5
  Demux : Demux  Outputs=[1 1 1 6]
  Ground : Ground
  Ground1 : Ground
  Mux : Mux  Inputs=2
  Mux1 : Mux  Inputs=[1 5 2 5]
  Product5 : Product  SaturateOnIntegerOverflow=on  RndMeth=Zero  InputSameDT=on  OutDataTypeStr=Inherit: Same as first input
  Sum : Sum  Inputs=-+  SaturateOnIntegerOverflow=on  InputSameDT=on  OutDataTypeStr=Inherit: Same as first input
  Sum1 : Sum  Inputs=+-  SaturateOnIntegerOverflow=on  InputSameDT=on  OutDataTypeStr=Inherit: Same as first input
  Sum2 : Sum  Inputs=--+  SaturateOnIntegerOverflow=on  InputSameDT=on  OutDataTypeStr=Inherit: Same as first input
  Terminator : Terminator
  Terminator1 : Terminator
  emission_in : Gain  Gain=emission_in  SaturateOnIntegerOverflow=on  OutDataTypeStr=Inherit: Same as input  ParamDataTypeStr=Inherit: Same as input
  surface of window : Gain  Gain=windowsurface  SaturateOnIntegerOverflow=on  OutDataTypeStr=Inherit: Same as input  ParamDataTypeStr=Inherit: Same as input
  surface of window glass : Gain  Gain=(1-frame)*windowsurface  SaturateOnIntegerOverflow=on  OutDataTypeStr=Inherit: Same as input  ParamDataTypeStr=Inherit: Same as input
  transmission_absorption : Subsystem
  u_convection : Gain  Gain=2.5  SaturateOnIntegerOverflow=on  OutDataTypeStr=Inherit: Same as input  ParamDataTypeStr=Inherit: Same as input
  u_rad : Constant  Value=5.6
  qdots2 : Outport
  "[S]" : Outport  Port=2
  wires:
  Ground1/1 -> Mux1/4
  Ground/1 -> Mux1/2
  Mux1/1 -> "[S]"/1
  Sum2/1 -> qdots2/1
  Demux/4 -> Terminator1/1
  "[AIV]"/1 -> Demux/1
  Demux/1 -> Terminator/1
  Mux/1 -> surface of window/1
  emission_in/1 -> Product5/1
  Sum1/1 -> Product5/2  "dTr"
  u_rad/1 -> emission_in/1
  Ts2/1 -> Sum/2, Sum1/1  "Ts"
  Product5/1 -> Mux/2, Sum2/2  "qdotr"
  u_convection/1 -> Sum2/1, Mux/1  "qdotc"
  "[sun_t]"/1 -> transmission_absorption/1(sun_t)
  surface of window glass/1 -> Mux1/1  "Qdot_sol"
  surface of window/1 -> Mux1/3  "[Qdotc, Qdotr]"
  Demux/2 -> Sum/1  "Tc"
  Sum/1 -> u_convection/1  "dTc"
  Demux/3 -> Sum1/2  "Tr"
  transmission_absorption/2(qdot_sol) -> surface of window glass/1  "qdot_sol (> =0)"
  transmission_absorption/1(qdot_abs) -> Sum2/3  "qabs"
  WDB/1 -> transmission_absorption/2(WDB)
  control/1 -> transmission_absorption/3(control)

== system carnot/Load/Houses/wall_floor/Window_with_Shading/lambda_window ==
  note: Timeconstant of window is calculated
      | in the mask initialization
  note: Heat conduction in a window (ONLY SURFACE LAYER CONNECTABLE)
  qdots1 : Inport
  qdots2 : Inport  Port=2
  Product1 : Product  SaturateOnIntegerOverflow=on  RndMeth=Zero  InputSameDT=on  OutDataTypeStr=Inherit: Same as first input
  Product6 : Product  SaturateOnIntegerOverflow=on  RndMeth=Zero  InputSameDT=on  OutDataTypeStr=Inherit: Same as first input
  R_win : Constant  Value=Rwin
  Sum1 : Sum  SaturateOnIntegerOverflow=on  InputSameDT=on  OutDataTypeStr=Inherit: Same as first input
  Sum3 : Sum  SaturateOnIntegerOverflow=on  InputSameDT=on  OutDataTypeStr=Inherit: Same as first input
  Transfer Fcn : TransferFcn  Denominator=[timeconst 1]
  Transfer Fcn1 : TransferFcn  Denominator=[timeconst 1]
  Ts1 : Outport
  Ts2 : Outport  Port=2
  wires:
  R_win/1 -> Product1/1, Product6/1  "R_win"
  Sum1/1 -> Transfer Fcn1/1
  Product1/1 -> Sum1/1
  Sum3/1 -> Transfer Fcn/1
  Product6/1 -> Sum3/1
  qdots2/1 -> Product1/2
  qdots1/1 -> Product6/2
  Transfer Fcn/1 -> Sum1/2, Ts1/1
  Transfer Fcn1/1 -> Sum3/2, Ts2/1

== system carnot/Source/Chiller/Absorption_Chiller_ddT/absorber // condenser/Tcooler_out ==
  T : Inport
  mdot : Inport  Port=2
  Qdot_E + Qdot_G : Inport  Port=3
  p : Inport  Port=4
  fluid : Inport  Port=5
  mix : Inport  Port=6
  Heat_Capacity : carnot/Basic/Material_Properties/Heat_Capacity  VariantControl=CarlibClassic  INPUTARGUMENTS=state variables (classic)  DEBUGLEVEL=DEBUGLEVEL  MAXTOTALWARNINGS=inf  MAXCONSECUTIVEWARNINGS=inf  WRITETOFILE=0  FILENAME='errors.txt'
  Product1 : Product  Inputs=//*  SaturateOnIntegerOverflow=on  InputSameDT=on  OutDataTypeStr=Inherit: Same as first input
  Saturation : Saturate  UpperLimit=inf  LowerLimit=1e-5
  Sum3 : Sum  SaturateOnIntegerOverflow=on  InputSameDT=on  OutDataTypeStr=Inherit: Same as first input
  Tcooler_out : Outport  InitialOutput=0
  wires:
  Qdot_E + Qdot_G/1 -> Product1/3
  Saturation/1 -> Product1/1
  Sum3/1 -> Tcooler_out/1
  mdot/1 -> Saturation/1
  Product1/1 -> Sum3/2
  Heat_Capacity/1 -> Product1/2
  T/1 -> Heat_Capacity/1, Sum3/1
  p/1 -> Heat_Capacity/2
  fluid/1 -> Heat_Capacity/3
  mix/1 -> Heat_Capacity/4

== system carnot/Source/Chiller/Absorption_Chiller_ddT/boiler/Qdot_G with deltadelta_t ==
  deltadelta_t : Inport
  Add1 : Sum
  Constant : Constant  Value=rG
  Gain1 : Gain  Gain=sG
  Transfer Fcn : TransferFcn  Denominator=[600 1]
  kW_2_W : Gain  Gain=1000
  Qdot_G [W] : Outport
  wires:
  Transfer Fcn/1 -> Qdot_G [W]/1
  kW_2_W/1 -> Transfer Fcn/1
  Add1/1 -> kW_2_W/1
  deltadelta_t/1 -> Gain1/1
  Gain1/1 -> Add1/2
  Constant/1 -> Add1/1

== system carnot/Source/Chiller/Absorption_Chiller_ddT/boiler/Thot_out ==
  Thot_in : Inport
  mdot : Inport  Port=2
  Qdot_G : Inport  Port=3
  p : Inport  Port=4
  fluid : Inport  Port=5
  mix : Inport  Port=6
  Heat_Capacity : carnot/Basic/Material_Properties/Heat_Capacity  VariantControl=CarlibClassic  INPUTARGUMENTS=state variables (classic)  DEBUGLEVEL=DEBUGLEVEL  MAXTOTALWARNINGS=inf  MAXCONSECUTIVEWARNINGS=inf  WRITETOFILE=0  FILENAME='errors.txt'
  Product1 : Product  Inputs=//*  SaturateOnIntegerOverflow=on  InputSameDT=on  OutDataTypeStr=Inherit: Same as first input
  Saturation : Saturate  UpperLimit=inf  LowerLimit=1e-5
  Sum3 : Sum  Inputs=+-  SaturateOnIntegerOverflow=on  InputSameDT=on  OutDataTypeStr=Inherit: Same as first input
  Thot_out : Outport  InitialOutput=0
  wires:
  Qdot_G/1 -> Product1/3
  Saturation/1 -> Product1/1
  Sum3/1 -> Thot_out/1
  mdot/1 -> Saturation/1
  Product1/1 -> Sum3/2
  Heat_Capacity/1 -> Product1/2
  Thot_in/1 -> Heat_Capacity/1, Sum3/1
  p/1 -> Heat_Capacity/2
  fluid/1 -> Heat_Capacity/3
  mix/1 -> Heat_Capacity/4

== system carnot/Source/Chiller/Absorption_Chiller_ddT/evaporator/Qdot_E with deltadelta_t ==
  deltadelta_t : Inport
  Add1 : Sum
  Constant : Constant  Value=rE
  Gain1 : Gain  Gain=sE
  Transfer Fcn : TransferFcn  Denominator=[600 1]
  kW_2_W : Gain  Gain=1000
  Qdot_E [W] : Outport
  wires:
  Transfer Fcn/1 -> Qdot_E [W]/1
  kW_2_W/1 -> Transfer Fcn/1
  Add1/1 -> kW_2_W/1
  deltadelta_t/1 -> Gain1/1
  Gain1/1 -> Add1/2
  Constant/1 -> Add1/1

== system carnot/Source/Chiller/Absorption_Chiller_ddT/evaporator/Tchilled_out ==
  note: Qdot_chilled_out = Qdot_chilled_in - Q_E
      | tchilled_out = Tchilled_in * mdot* cp - Qdot_E / (mdot * cp)
  T : Inport
  mdot : Inport  Port=2
  Qdot_E : Inport  Port=3
  p : Inport  Port=4
  fluid : Inport  Port=5
  mix : Inport  Port=6
  Heat_Capacity : carnot/Basic/Material_Properties/Heat_Capacity  VariantControl=CarlibClassic  INPUTARGUMENTS=state variables (classic)  DEBUGLEVEL=DEBUGLEVEL  MAXTOTALWARNINGS=inf  MAXCONSECUTIVEWARNINGS=inf  WRITETOFILE=0  FILENAME='errors.txt'
  Product1 : Product  Inputs=//*  SaturateOnIntegerOverflow=on  InputSameDT=on  OutDataTypeStr=Inherit: Same as first input
  Saturation : Saturate  UpperLimit=inf  LowerLimit=1e-5
  Sum3 : Sum  Inputs=+-  SaturateOnIntegerOverflow=on  InputSameDT=on  OutDataTypeStr=Inherit: Same as first input
  Tcold : Outport  InitialOutput=0
  wires:
  Product1/1 -> Sum3/2
  Qdot_E/1 -> Product1/3
  mdot/1 -> Saturation/1
  Saturation/1 -> Product1/1
  Sum3/1 -> Tcold/1
  Heat_Capacity/1 -> Product1/2
  T/1 -> Heat_Capacity/1, Sum3/1
  p/1 -> Heat_Capacity/2
  fluid/1 -> Heat_Capacity/3
  mix/1 -> Heat_Capacity/4

== system carnot/Source/Chiller/Compression_Air_Water_Chiller/Lookup_tables _COP + Q_cold_faktor/runtime_AC ==
  control_AC : Inport
  Integrator : Integrator  ExternalReset=either  InitialCondition=1
  runtime : Outport
  wires:
  control_AC/1 -> Integrator/2, Integrator/1
  Integrator/1 -> runtime/1

== system carnot/Source/Chiller/Cooling_Tower/Feuchtkugel- temperatureinfluss // wet-bulb temperature effect/Abgleich  ==
  note: Durch den Abgleich der vorliegenden Datensätze
      | wierd die Annahme getroffen
      | das bei einer reduzierung der Feuchtkugeltemp um 1K
      |  sich die Kaltwassertemp um 0.27K sinkt.
      |
      | y = ((t_FK-15)*0.27)+t_ia_100
      |
      | Ab eine Eintritstemperatur von 41 °C wierd mit
      | dem Faktor 0,25 K gerechnet.
      |
      | y = ((t_FK-15)*0.25)+t_ia_100
  t_FK : Inport
  t_ie : Inport  Port=2
  t_ia_FK15 : Inport  Port=3
  Embedded MATLAB Function : MATLAB Function  TreatAsAtomicUnit=on
  t_ia_FK : Outport
  wires:
  Embedded MATLAB Function/1(y) -> t_ia_FK/1
  t_FK/1 -> Embedded MATLAB Function/1(t_fk)
  t_ia_FK15/1 -> Embedded MATLAB Function/2(t_ia_fk15)
  t_ie/1 -> Embedded MATLAB Function/3(t_ie)

== system carnot/Source/Chiller/Cooling_Tower/Feuchtkugel- temperatureinfluss // wet-bulb temperature effect/wet-bulb 15 °C ==
  t_ie : Inport
  Lookup Table : Lookup  InputValues=[26 28 30 32 34 36 38 40 42 44 79.2]  Table=[22.6 23.9 25.2 26.4 27.7 28.9 30.1 31.2 32.4 33.5 49.25]
  t_ia_FK15 : Outport
  wires:
  t_ie/1 -> Lookup Table/1
  Lookup Table/1 -> t_ia_FK15/1

== system carnot/Source/Chiller/Cooling_Tower/Leistungseinflüsse // influence on coolingpower/Qdot_i_FK ==
  t_ia_FK : Inport
  t_ie : Inport  Port=2
  Fluid_Type : Inport  Port=3
  Add : Sum
  Constant : Constant  Value=0.3
  Constant1 : Constant  Value=2.4
  Constant2 : Constant  Value=2
  Density : carnot/Basic/Material_Properties/Density  VariantControl=CarlibClassic  INPUTARGUMENTS=state variables (classic)  DEBUGLEVEL=DEBUGLEVEL  MAXTOTALWARNINGS=inf  MAXCONSECUTIVEWARNINGS=inf  WRITETOFILE=0  FILENAME='errors.txt'
  Divide1 : Product  Inputs=*/
  Divide2 : Product  Inputs=*/
  Divide3 : Product  Inputs=*/
  Heat_Capacity : carnot/Basic/Material_Properties/Heat_Capacity  VariantControl=CarlibClassic  INPUTARGUMENTS=state variables (classic)  DEBUGLEVEL=DEBUGLEVEL  MAXTOTALWARNINGS=inf  MAXCONSECUTIVEWARNINGS=inf  WRITETOFILE=0  FILENAME='errors.txt'
  Product : Product  Inputs=4  RndMeth=Zero
  Subtract : Sum  Inputs=+-
  phi_Le1 : Constant  Value=1000
  phi_Le2 : Constant  Value=1000
  phi_Le3 : Constant  Value=1e5
  Qdot_i_FK : Outport
  wires:
  t_ia_FK/1 -> Subtract/2, Add/2
  Product/1 -> Qdot_i_FK/1
  Subtract/1 -> Product/1
  t_ie/1 -> Density/1, Subtract/1, Add/1
  Constant/1 -> Heat_Capacity/4, Density/4
  Density/1 -> Divide2/1
  phi_Le3/1 -> Heat_Capacity/2, Density/2
  Fluid_Type/1 -> Heat_Capacity/3, Density/3
  phi_Le1/1 -> Divide2/2
  Divide2/1 -> Product/4
  Constant1/1 -> Product/3
  Heat_Capacity/1 -> Divide3/1
  Constant2/1 -> Divide1/2
  Divide1/1 -> Heat_Capacity/1
  Add/1 -> Divide1/1
  phi_Le2/1 -> Divide3/2
  Divide3/1 -> Product/2

== system carnot/Source/Chiller/Cooling_Tower/Leistungseinflüsse // influence on coolingpower/Qdot_i_ist  ==
  Qdot_i_FK : Inport
  n_Fan [%] : Inport  Port=2
  Fluid_mix : Inport  Port=3
  mdot_i : Inport  Port=4
  Fluid_Type : Inport  Port=5
  t_ie : Inport  Port=6
  Constant : Constant  Value=92
  Constant2 : Constant  Value=100
  Density : carnot/Basic/Material_Properties/Density  VariantControl=CarlibClassic  INPUTARGUMENTS=state variables (classic)  DEBUGLEVEL=DEBUGLEVEL  MAXTOTALWARNINGS=inf  MAXCONSECUTIVEWARNINGS=inf  WRITETOFILE=0  FILENAME='errors.txt'
  Divide : Product  Inputs=**/
  Divide1 : Product  Inputs=*/
  Divide2 : Product  Inputs=*/
  Lookup Table (2-D) Volumenstromänderung : Lookup2D  RowIndex=[1.07 1.77 2.4 2.65 3.03]  ColumnIndex=[25 30 35 40 45 50 55 60 65]  Table=[0.7248 0.7054 0.6860 0.6666 0.6472 0.6278 0.6084 0.5890 0.5696; 0.9493 0.9294 0.9096 0.8897 0.8698 0.8500 0.8301 0.8103 0.7904; 1 1 1 1 1 1 1 1 1; 1.1191 1.1295 1.0956 1.0674 1.0450 1.0284 1.0175 1.0123 1.0129; 1.2370 1.1910 1.1526 1.1219 1.0988 1.0833 1.0754 1.0752 1.0826]
  Lookup Table Lüfterdrehzahl : Lookup  InputValues=[0 0.2 0.3 0.5 0.7 0.9 1]  Table=[0 0.37 0.482 0.625 0.786 0.928 1]
  Lookup Table1 Glykol : Lookup  InputValues=[0 0.1 0.2 0.3 0.4 0.5 0.6 0.7 0.8 0.9 1]  Table=[1 0.98 0.95 0.92 0.875 0.83 0.78 0.73 0.68 0.63 0.57]
  Product : Product  RndMeth=Zero
  Product1 : Product  RndMeth=Zero
  Product2 : Product  RndMeth=Zero
  phi_Le1 : Constant  Value=1000
  phi_Le3 : Constant  Value=1e5
  Qdot_i_ist : Outport
  wires:
  n_Fan [%]/1 -> Lookup Table Lüfterdrehzahl/1
  Lookup Table Lüfterdrehzahl/1 -> Product/2
  Qdot_i_FK/1 -> Product/1
  Product/1 -> Divide/1
  Product1/1 -> Product2/1
  Lookup Table1 Glykol/1 -> Product2/2
  Fluid_mix/1 -> Density/4, Lookup Table1 Glykol/1
  Divide/1 -> Product1/1
  Constant/1 -> Divide/3
  mdot_i/1 -> Divide1/1
  Product2/1 -> Qdot_i_ist/1
  Density/1 -> Divide2/1
  phi_Le3/1 -> Density/2
  Fluid_Type/1 -> Density/3
  phi_Le1/1 -> Divide2/2
  Divide2/1 -> Divide1/2
  t_ie/1 -> Density/1, Lookup Table (2-D) Volumenstromänderung/2  "column"
  Divide1/1 -> Lookup Table (2-D) Volumenstromänderung/1  "row"
  Lookup Table (2-D) Volumenstromänderung/1 -> Product1/2
  Constant2/1 -> Divide/2

== system carnot/Source/Chiller/Cooling_Tower/Leistungseinflüsse // influence on coolingpower/t_ia_ist  ==
  Qdot_i_ist : Inport
  t_ie : Inport  Port=2
  cp_i : Inport  Port=3
  mdot : Inport  Port=4
  Add : Sum  Inputs=-+
  Divide : Product  Inputs=*//
  Divide1 : Product  Inputs=*/
  isinf : MATLAB Function  TreatAsAtomicUnit=on
  isnan : MATLAB Function  TreatAsAtomicUnit=on
  phi_Le2 : Constant  Value=1000
  t_ia_ist : Outport
  wires:
  Add/1 -> t_ia_ist/1
  Qdot_i_ist/1 -> Divide/1
  t_ie/1 -> Add/2
  Divide/1 -> isnan/1(u)
  cp_i/1 -> Divide1/1
  isnan/1(y) -> isinf/1(u)
  phi_Le2/1 -> Divide1/2
  Divide1/1 -> Divide/2
  mdot/1 -> Divide/3
  isinf/1(y) -> Add/1

== system carnot/Source/Chiller/Cooling_Tower/Verbrauch // consumption/Strom ==
  control_Fan : Inport
  P_Fan : Inport  Port=2
  Add : Sum
  Integrator1 : Integrator
  Product : Product  RndMeth=Zero
  Product2 : Product  Inputs=*/  SaturateOnIntegerOverflow=on  RndMeth=Zero  InputSameDT=on  OutDataTypeStr=Inherit: Same as first input
  Rieselwasserpumpe [kW] : Constant  Value=0.25
  factor1 : Constant  Value=3600
  energy : Outport
  power : Outport  Port=2
  wires:
  Rieselwasserpumpe [kW]/1 -> Add/1
  Product/1 -> power/1, Integrator1/1
  control_Fan/1 -> Product/1
  Add/1 -> Product/2
  P_Fan/1 -> Add/2
  Integrator1/1 -> Product2/1
  factor1/1 -> Product2/2
  Product2/1 -> energy/1

== system carnot/Source/Chiller/Cooling_Tower/Verbrauch // consumption/Verdunstung ==
  control_Fan : Inport
  t_le : Inport  Port=2
  phi_le : Inport  Port=3
  Vdot_Fan : Inport  Port=4
  Qdot : Inport  Port=5
  t_ie : Inport  Port=6
  "Enthalpie " : Subsystem
  Integrator1 : Integrator
  Product : Product  RndMeth=Zero
  Product1 : Product  RndMeth=Zero
  Product2 : Product  Inputs=*/  SaturateOnIntegerOverflow=on  RndMeth=Zero  InputSameDT=on  OutDataTypeStr=Inherit: Same as first input
  Product3 : Product  RndMeth=Zero
  RelHum2x : carnot/Basic/Material_Properties/RelHum2x
  Saturation_Temperature : carnot/Basic/Material_Properties/Saturation_Temperature  VariantControl=CarlibClassic  INPUTARGUMENTS=state variables (classic)  DEBUGLEVEL=WARNINGLEVEL  MAXTOTALMESSAGES=inf  MAXCONSECUTIVEMESSAGES=inf  WRITETOFILE=0  FILENAME='errors.txt'
  Verdunstungsmenge : MATLAB Function  TreatAsAtomicUnit=on
  air : Constant  Value=2
  factor1 : Constant  Value=3600
  p : Constant  Value=1e5
  roh_air : Constant  Value=1.29
  Wasserverbrauch : Outport
  wires:
  t_le/1 -> RelHum2x/1, Saturation_Temperature/1, "Enthalpie "/2(t_le)
  p/1 -> RelHum2x/2, Saturation_Temperature/2, Verdunstungsmenge/7(p)
  phi_le/1 -> RelHum2x/3
  Vdot_Fan/1 -> Product/1
  roh_air/1 -> Product/2
  "Enthalpie "/1(h_le) -> Verdunstungsmenge/1(h_le)
  RelHum2x/1 -> "Enthalpie "/1(x_le), Saturation_Temperature/4, Verdunstungsmenge/5(x_le)
  Qdot/1 -> Verdunstungsmenge/3(qdot)
  Saturation_Temperature/1 -> Verdunstungsmenge/6(t_tau)
  air/1 -> Saturation_Temperature/3
  Integrator1/1 -> Product2/1
  factor1/1 -> Product2/2
  Product2/1 -> Wasserverbrauch/1
  Product1/1 -> Integrator1/1
  control_Fan/1 -> Product1/1
  Product3/1 -> Product1/2
  Product/1 -> Verdunstungsmenge/2(mdot), Product3/1
  t_ie/1 -> Verdunstungsmenge/4(t_ie)
  Verdunstungsmenge/1(x_fl) -> Product3/2

== system carnot/Source/Heat_Pump/Ground_Source_Heat_Exchanger/Randbedingung 2/g-function ==
  note: Trichter: 1/(4*pi*lambdaErde)
  T(i,1)-T(i,0) : Inport
  Constant : Constant  Value=t_start
  Dd1 : Gain  Gain=L1/(Ts_Trichter*Dl)  SaturateOnIntegerOverflow=on  OutDataTypeStr=Inherit: Same as input  ParamDataTypeStr=Inherit: Same as input
  Dd2 : Gain  Gain=1/(2*pi*lambdaErde)  SaturateOnIntegerOverflow=on  OutDataTypeStr=Inherit: Same as input  ParamDataTypeStr=Inherit: Same as input
  Digital Clock : DigitalClock
  Integrator : Integrator  ExternalReset=rising
  Product : Product  SaturateOnIntegerOverflow=on  RndMeth=Zero  InputSameDT=on  OutDataTypeStr=Inherit: Same as first input
  Pulse Generator : DiscretePulseGenerator  PulseType=Time based  Period=Ts_Trichter  PulseWidth=50  PhaseDelay=300
  RechenRadius : Constant  Value=Rechenradius  VectorParams1D=off
  Sum : Sum  Inputs=|+-  SaturateOnIntegerOverflow=on  InputSameDT=on  OutDataTypeStr=Inherit: Same as first input
  Sum1 : Sum  Inputs=++|  SaturateOnIntegerOverflow=on  InputSameDT=on  OutDataTypeStr=Inherit: Same as first input
  Sum4 : Sum  Inputs=|++  SaturateOnIntegerOverflow=on  InputSameDT=on  OutDataTypeStr=Inherit: Same as first input
  Unit Delay : UnitDelay
  Unit Delay1 : UnitDelay
  Zero-Order Hold2 : ZeroOrderHold
  Zero-Order Hold3 : ZeroOrderHold
  g-function : Lookup2D  RowIndex=t_Trichter  ColumnIndex=r_Trichter  Table=gfunction  SaturateOnIntegerOverflow=on  InputSameDT=on
  DeltaT : Outport
  wires:
  T(i,1)-T(i,0)/1 -> Integrator/1
  Zero-Order Hold2/1 -> Sum/1, Unit Delay/1
  Zero-Order Hold3/1 -> g-function/2
  Sum4/1 -> DeltaT/1, Unit Delay1/1
  Unit Delay1/1 -> Sum4/2
  Dd2/1 -> Product/2
  Product/1 -> Sum4/1
  RechenRadius/1 -> Zero-Order Hold3/1
  g-function/1 -> Dd2/1
  Sum/1 -> Product/1
  Unit Delay/1 -> Sum/2
  Dd1/1 -> Zero-Order Hold2/1
  Integrator/1 -> Dd1/1
  Pulse Generator/1 -> Integrator/2
  Digital Clock/1 -> Sum1/2
  Sum1/1 -> g-function/1
  Constant/1 -> Sum1/1
